simulink model "recv_cmd"  (R2021a)
settings: Solver=FixedStepAuto  StartTime=0.0  StopTime=inf  RelTol=1e-3
libraries: slrealtimesharedmemorylib x5, simulink x4, slrealtimeutilitieslib x1, slrealtimeiplib x1
settings Model: OrderedModelArguments=off  Creator=Ruixuan  LastModifiedBy=Ruixuan
settings SolverCC: ConcurrentTasks=on  PositivePriorityOrder=on  AutoInsertRateTranBlk=on  InsertRTBMode=Never (minimum delay)
settings OptimizationCC: BlockReduction=off  DefaultParameterBehavior=Inlined  OptimizeBlockIOStorage=off
settings DebuggingCC: TasksWithSamePriorityMsg=none
settings HardwareCC: ProdBitPerLong=64  ProdLongLongMode=on  ProdHWDeviceType=Intel->x86-64 (Linux 64)
settings ModelReferenceCC: ModelReferenceNumInstancesAllowed=Single
settings RTWCC: Description=Simulink Real-Time  SystemTargetFile=slrealtime.tlc  TemplateMakefile=slrealtime_default_tmf  Toolchain=Simulink Real-Time Toolchain  BuildConfiguration=Faster Runs  CodeExecutionProfiling=on  TargetLang=C++

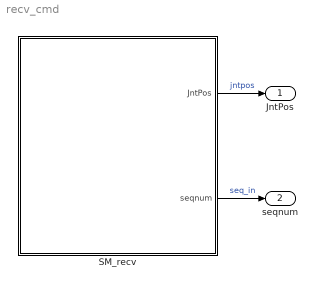
== system recv_cmd ==
  SM_recv : Subsystem  Priority=1  mask(StreamMotion_receive){}
  JntPos : Outport  VectorParamsAs1DForOutWhenUnconnected=off
  seqnum : Outport  Port=2  VectorParamsAs1DForOutWhenUnconnected=off
  wires:
  SM_recv/1(JntPos) -> JntPos/1  "jntpos"
  SM_recv/2(seqnum) -> seqnum/1  "seq_in"

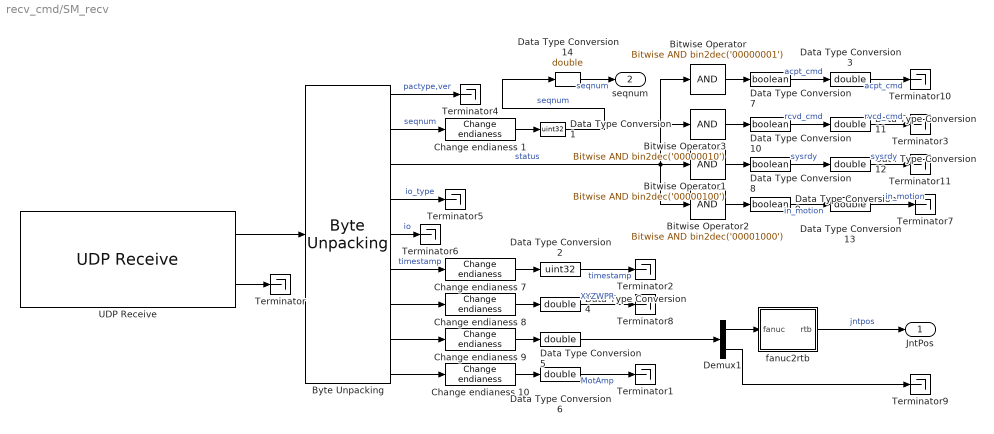
== system recv_cmd/SM_recv ==
  Bitwise Operator : simulink/Logic and Bit Operations/Bitwise Operator  logicop=AND  UseBitMask=on  BitMask=bin2dec('00000001')  BitMaskRealWorld=Stored Integer
  Bitwise Operator1 : simulink/Logic and Bit Operations/Bitwise Operator  logicop=AND  UseBitMask=on  BitMask=bin2dec('00000100')  BitMaskRealWorld=Stored Integer
  Bitwise Operator2 : simulink/Logic and Bit Operations/Bitwise Operator  logicop=AND  UseBitMask=on  BitMask=bin2dec('00001000')  BitMaskRealWorld=Stored Integer
  Bitwise Operator3 : simulink/Logic and Bit Operations/Bitwise Operator  logicop=AND  UseBitMask=on  BitMask=bin2dec('00000010')  BitMaskRealWorld=Stored Integer
  "Byte Unpacking " : slrealtimeutilitieslib/Byte Unpacking  Priority=4  MaskUnpackedDataTypes={['uint32'],'uint32','uint8','uint8',['uint16'],'uint32',['single'],['single'],['single']}  MaskUnpackedDataSizes={[2],[1],[1],[1],[3],[1],[9],[9],[9]}  MaskAlignment=1
      settings: SourceProductBaseCode=XP
  Change endianess {1,8..10} (4 alike) : slrealtimesharedmemorylib/Change endianess  numInp=1  lengthIn=Byte
      settings: SourceProductBaseCode=XP
  Change endianess 7 : slrealtimesharedmemorylib/Change endianess  Priority=15  numInp=1  lengthIn=Byte
      settings: SourceProductBaseCode=XP
  Data Type Conversion1 : DataTypeConversion  OutDataTypeStr=uint32
  Data Type Conversion{7..10} (4 alike) : DataTypeConversion  OutDataTypeStr=boolean
  Data Type Conversion{3..6,11..14} (8 alike) : DataTypeConversion  OutDataTypeStr=double
  Data Type Conversion2 : DataTypeConversion  OutDataTypeStr=uint32
  Demux1 : Demux  Outputs=[6,3]
  Terminator{,1..11} (12 alike) : Terminator
  UDP Receive : slrealtimeiplib/UDP Receive  Priority=3  useHostTargetConn=off  ipAddress=192.168.1.101  localPort=60015  rcvWidth=132  rcvFmAny=off  fmAddress=192.168.1.100  sampleTime=Ts
      settings: SourceProductBaseCode=XP
  fanuc2rtb : Subsystem  mask(FANUC2RTB){}
      mask help: type convention from fanuc style joint position to robotic toolbox style joint position
  JntPos : Outport  VectorParamsAs1DForOutWhenUnconnected=off
  seqnum : Outport  Port=2  VectorParamsAs1DForOutWhenUnconnected=off
  wires:
  Bitwise Operator/1 -> Data Type Conversion7/1
  Bitwise Operator2/1 -> Data Type Conversion9/1
  Change endianess 7/1 -> Data Type Conversion2/1
  "Byte Unpacking "/1 -> Terminator4/1  "pactype,ver"
  "Byte Unpacking "/6 -> Change endianess 7/1  "timestamp"
  Data Type Conversion7/1 -> Data Type Conversion3/1  "acpt_cmd"
  UDP Receive/1 -> "Byte Unpacking "/1
  Data Type Conversion3/1 -> Terminator10/1  "acpt_cmd"
  Change endianess 1/1 -> Data Type Conversion1/1
  "Byte Unpacking "/4 -> Terminator5/1  "io_type"
  fanuc2rtb/1(rtb) -> JntPos/1  "jntpos"
  Bitwise Operator3/1 -> Data Type Conversion10/1
  Bitwise Operator1/1 -> Data Type Conversion8/1
  UDP Receive/2 -> Terminator/1
  "Byte Unpacking "/2 -> Change endianess 1/1  "seqnum"
  Demux1/2 -> Terminator9/1
  "Byte Unpacking "/7 -> Change endianess 8/1
  "Byte Unpacking "/9 -> Change endianess 10/1
  Data Type Conversion13/1 -> Terminator7/1  "in_motion"
  "Byte Unpacking "/8 -> Change endianess 9/1
  Data Type Conversion6/1 -> Terminator1/1  "MotAmp"
  Data Type Conversion2/1 -> Terminator2/1  "timestamp"
  Data Type Conversion1/1 -> Data Type Conversion14/1  "seqnum"
  Data Type Conversion14/1 -> seqnum/1  "seqnum"
  Data Type Conversion10/1 -> Data Type Conversion11/1  "rcvd_cmd"
  Change endianess 8/1 -> Data Type Conversion4/1
  Data Type Conversion5/1 -> Demux1/1
  Data Type Conversion11/1 -> Terminator3/1  "rvcd_cmd"
  Change endianess 9/1 -> Data Type Conversion5/1
  Data Type Conversion8/1 -> Data Type Conversion12/1  "sysrdy"
  Change endianess 10/1 -> Data Type Conversion6/1
  "Byte Unpacking "/5 -> Terminator6/1  "io"
  "Byte Unpacking "/3 -> Bitwise Operator1/1, Bitwise Operator3/1, Bitwise Operator/1, Bitwise Operator2/1  "status"
  Data Type Conversion9/1 -> Data Type Conversion13/1  "in_motion"
  Data Type Conversion4/1 -> Terminator8/1  "XYZWPR"
  Data Type Conversion12/1 -> Terminator11/1  "sysrdy"
  Demux1/1 -> fanuc2rtb/1(fanuc)

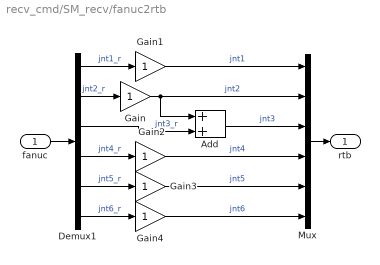
== system recv_cmd/SM_recv/fanuc2rtb ==
  fanuc : Inport
  Add : Sum
  Demux1 : Demux  Outputs=6
  Gain{,1..4} (5 alike) : Gain
  Mux : Mux  Inputs=6
  rtb : Outport  VectorParamsAs1DForOutWhenUnconnected=off
  wires:
  Demux1/3 -> Add/2  "jnt3_r"
  Demux1/2 -> Gain/1  "jnt2_r"
  Gain/1 -> Mux/2, Add/1  "jnt2"
  Add/1 -> Mux/3  "jnt3"
  Demux1/6 -> Gain4/1  "jnt6_r"
  Demux1/1 -> Gain1/1  "jnt1_r"
  Demux1/5 -> Gain3/1  "jnt5_r"
  Demux1/4 -> Gain2/1  "jnt4_r"
  Mux/1 -> rtb/1
  fanuc/1 -> Demux1/1
  Gain1/1 -> Mux/1  "jnt1"
  Gain2/1 -> Mux/4  "jnt4"
  Gain3/1 -> Mux/5  "jnt5"
  Gain4/1 -> Mux/6  "jnt6"
